simulink model "QpskSineMod23"  (R2024a)
settings: Solver=VariableStepAuto  StartTime=0.0  StopTime=10.0  RelTol=1e-3
model workspace (MAT data in the model file):
  samp = 10
libraries: commdigbbndpm3 x2, commchan3 x1, commrandsrc3 x1
settings Model: Creator=Avinash  LastModifiedBy=Avinash

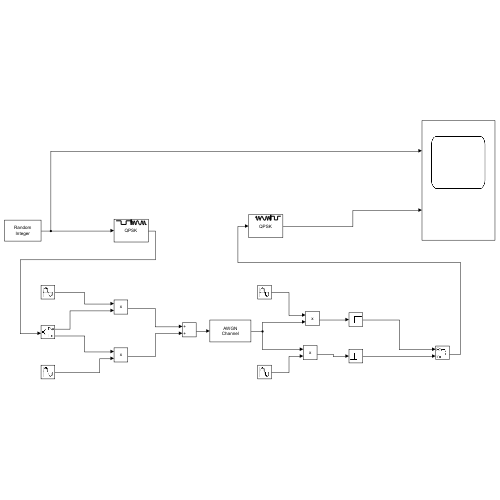
[thumbnail: Simulink's stored preview of the top-level diagram]
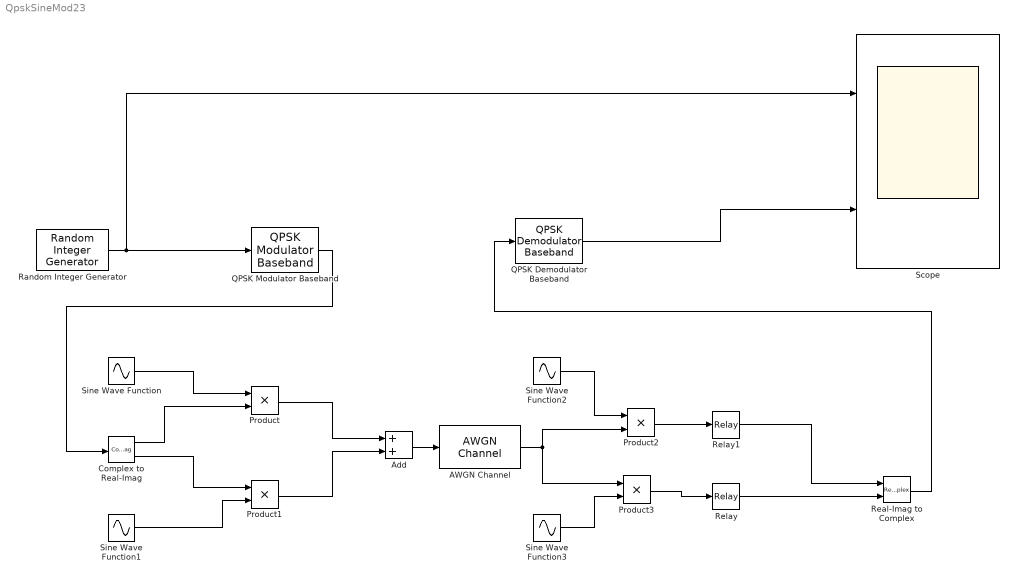
== system QpskSineMod23 ==
  AWGN Channel : commchan3/AWGN Channel  LegacyMode=off  NoiseMethod="Signal to noise ratio  (SNR)"  noiseMode="Signal to noise ratio  (SNR)"  EbNo=10  EsNo=10  SNR=35  BitsPerSymbol=1  SignalPower=1  SamplesPerSymbol=1  SymbolPeriod=1  VarianceSource=Parameter  Variance=1  RandomStream=Global stream  Seed=67  SimulateUsing=Code generation
  Add : Sum
  Complex to Real-Imag : ComplexToRealImag
  Product{,1..3} (4 alike) : Product
  QPSK Demodulator Baseband : commdigbbndpm3/QPSK Demodulator Baseband  OutType=Integer  DecType=Hard decision  VarSource=Dialog  Variance=1  Dec=Gray  Ph=pi/4  outDtype1=Inherit via internal rule  outDtype2=Inherit via internal rule  derotateFactorWordLen=16  derotateFactorDataTypeStr=Inherit: Same word length as input  derotateFactorLastDataTypeStr=Inherit: Same word length as input
  QPSK Modulator Baseband : commdigbbndpm3/QPSK Modulator Baseband  InType=Integer  Enc=Gray  Ph=pi/4  outDtype=double  outWordLen=16  outUDDataType=sfix(16)  outFracLenMode=Best precision  outFracLen=15  outDataTypeStr=double  outLastDataTypeStr=double
  Random Integer Generator : commrandsrc3/Random Integer Generator  SetSize=4  SeedSource=Auto  Seed=0  SampleTime=1  SamplesPerFrame=1  OutputDataType=double  SimulateUsing=Interpreted execution
  Real-Imag to Complex : RealImagToComplex
  Relay : Relay  OnSwitchValue=15  OffSwitchValue=-15  OnOutputValue=1/2^0.5  OffOutputValue=-1/2^0.5
  Relay1 : Relay  OnSwitchValue=15  OffSwitchValue=-15  OnOutputValue=1/2^0.5  OffOutputValue=-1/2^0.5
  Scope : Scope  NumInputPorts=2
  Sine Wave Function : Sin  Amplitude=samp  Frequency=4*2*pi  Phase=pi/2  SampleTime=0.001
  Sine Wave Function1 : Sin  Amplitude=samp  Frequency=4*2*pi  SampleTime=0.001
  Sine Wave Function2 : Sin  Amplitude=samp  Frequency=4*2*pi  Phase=pi/2  SampleTime=0.001
  Sine Wave Function3 : Sin  Amplitude=samp  Frequency=4*2*pi  SampleTime=0.001
  wires:
  Random Integer Generator/1 -> QPSK Modulator Baseband/1, Scope/1
  QPSK Modulator Baseband/1 -> Complex to Real-Imag/1
  Sine Wave Function/1 -> Product/1
  Complex to Real-Imag/1 -> Product/2
  Complex to Real-Imag/2 -> Product1/1
  Sine Wave Function1/1 -> Product1/2
  Product1/1 -> Add/2
  Product/1 -> Add/1
  Sine Wave Function2/1 -> Product2/1
  Sine Wave Function3/1 -> Product3/2
  Product2/1 -> Relay1/1
  Product3/1 -> Relay/1
  Relay/1 -> Real-Imag to Complex/2
  Relay1/1 -> Real-Imag to Complex/1
  QPSK Demodulator Baseband/1 -> Scope/2
  Real-Imag to Complex/1 -> QPSK Demodulator Baseband/1
  Add/1 -> AWGN Channel/1
  AWGN Channel/1 -> Product3/1, Product2/2
